simulink model "QD_V2"  (R2019a)
settings: Solver=ode4  StartTime=0  StopTime=10  FixedStep=0.001  RelTol=1e-3  EnableMultiTasking=on
model workspace (MAT data in the model file):
  ChStern = 20.5517740291
  CvStern = 205.517740291
  StartTime = '0'
  StopTime = '100'
  c = 0
  deltaControlled = 0
  deltaH = [0 0.02 0.04 0.06 0.08 0.1 0.12 0.14 0.16 0.18 0.2 0.22 0.24 0.26 0.28 0.3 0.32 0.34 0.36 0.38 0.4 0.42 0.44 0.46 0.48 0.5 0.52 0.54 0.56 0.58 0.6 0.62 0.64 0.66 0.68 0.7 0.72 0.74 0.76 0.78 0.8 0.82 0.84 0.86 0.88 0.9 0.92 0.94 0.96 0.98 1 1.02 1.04 1.06 1.08 1.1 1.12 1.14 1.16 1.18 1.2 1.22 1.24 1.26 1.28 1.3 1.32 1.34 1.36 1.38 1.4 1.42 1.44 1.46 1.48 1.5 1.52 1.54 1.56 1.58 1.6 1.62 1.64 1.66 1.68 1.7 1.72 1.74 1.76 1.78 1.8 1.82 1.84 1.86 1.88 1.9 1.92 1.94 1.96 1.98 2 2.02 2.04 2.06 2.08 2.1 2.12 2.14 2.16 2.18 2.2 2.22 2.24 2.26 2.28 2.3 2.32 2.34 2.36 2.38 2.4 2.42 2.44 2.46 2.48 2.5 2.52 2.54 2.56 2.58 2.6 2.62 2.64 2.66 2.68 2.7 2.72 2.74 2.76 2.78 2.8 2.82 2.84 2.86 2.88 2.9 2.92 2.94 2.96 2.98 3 3.02 3.04 3.06 3.08 3.1 3.12 3.14 3.16 3.18 3.2 3.22 3.24 3.26 3.28 3.3 3.32 3.34 3.36 3.38 3.4 3.42 3.44 3.46 3.48 3.5 3.52 3.54 3.56 3.58 3.6 3.62 3.64 3.66 3.68 3.7 3.72 3.74 3.76 3.78 3.8 3.82 3.84 3.86 3.88 3.9 3.92 3.94 3.96 3.98 4 4.02 4.04 4.06 4.08 4.1 4.12 4.14 4.16 4.18 4.2 4.22 4.24 4.26 4.28 4.3 4.32 4.34 4.36 4.38 4.4 4.42 4.44 4.46 4.48 4.5 4.52 4.54 4.56 4.58 4.6 4.62 4.64 4.66 4.68 4.7 4.72 4.74 4.76 4.78 4.8 4.82 4.84 4.86 4.88 4.9 4.92 4.94 4.96 4.98 5 5.02 5.04 5.06 5.08 5.1 5.12 5.14 5.16 5.18 5.2 5.22 5.24 5.26 5.28 5.3 5.32 5.34 5.36 5.38 5.4 5.42 5.44 5.46 5.48 5.5 5.52 5.54 5.56 5.58 5.6 5.62 5.64 5.66 5.68 5.7 5.72 5.74 5.76 5.78 5.8 5.82 5.84 5.86 5.88 5.9 5.92 5.94 5.96 5.98 6]
  g = 9.81
  is = 16
  lh = 1.45
  lv = 1.35
  m = 1550
  mDivTheta = 0.553571428571
  rSoll = 1
  theta = 2800
  v = 50
  x0 = 0
libraries: simulink x1
settings Model: Creator=tmonn  LastModifiedBy=Felix
settings DataIOCC: ExternalInput=c  ReturnWorkspaceOutputs=off
settings OptimizationCC: LifeSpan=inf
settings DebuggingCC: UnderspecifiedInitializationDetection=Classic  MergeDetectMultiDrivingBlocksExec=none  SFUnexpectedBacktrackingDiag=warning  SFNoUnconditionalDefaultTransitionDiag=warning  SFExecutionAtInitializationDiag=none  UnderSpecifiedDimensionMsg=warning  ArithmeticOperatorsInVariantConditions=warning
settings SFSimCC: SimUseLocalCustomCode=off
settings RTWCC: RTWUseLocalCustomCode=off
settings CodeAppCC: StateflowObjectComments=on
settings GRTTargetCC: TargetLangStandard=C89/C90 (ANSI)  GeneratePreprocessorConditionals=Disable all
settings ConfigComp: CovMetricSettings=dw  CovHtmlReporting=on  CovSaveCumulativeToWorkspaceVar=on  CovSaveSingleToWorkspaceVar=on  CovExternalEMLEnable=off

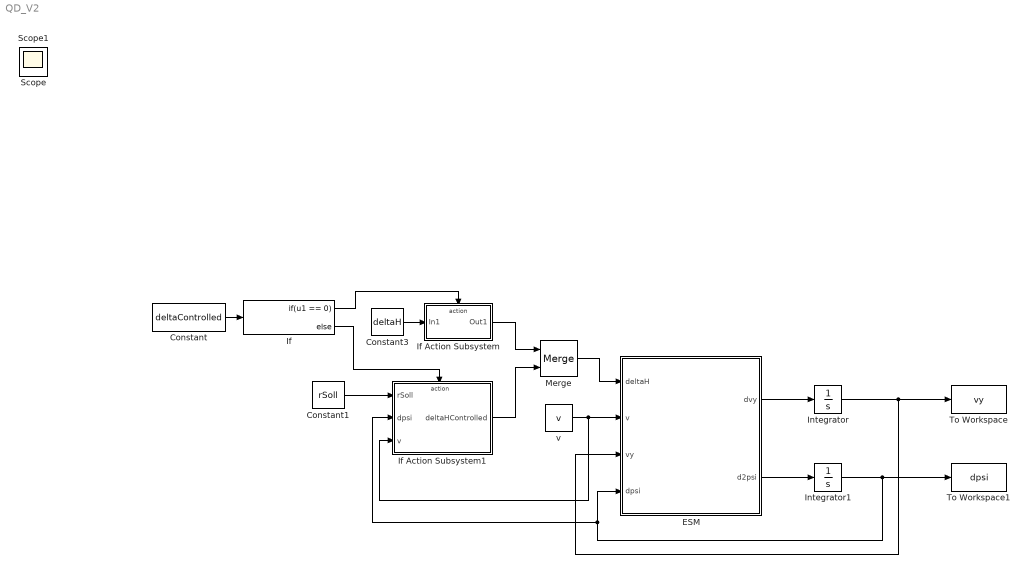
== system QD_V2 ==
  Constant : Constant  Value=deltaControlled
  Constant1 : Constant  Value=rSoll
  Constant3 : Constant  Value=deltaH
  ESM : Subsystem
  If : If  IfExpression=u1 == 0
  If Action Subsystem : Subsystem  TreatAsAtomicUnit=on
  If Action Subsystem1 : Subsystem  TreatAsAtomicUnit=on
  Integrator : Integrator
  Integrator1 : Integrator
  Merge : Merge  AllowUnequalInputPortWidths=on
  To Workspace : ToWorkspace  VariableName=vy  SaveFormat=Timeseries  SampleTime=-1
  To Workspace1 : ToWorkspace  VariableName=dpsi  SaveFormat=Timeseries  SampleTime=-1
  v : Constant  Value=v
  Scope : Scope
  Scope1 : Scope
  wires:
  ESM/1(dvy) -> Integrator/1
  ESM/2(d2psi) -> Integrator1/1
  Integrator/1 -> To Workspace/1, ESM/3(vy)
  If Action Subsystem/1(Out1) -> Merge/1
  Constant1/1 -> If Action Subsystem1/1(rSoll)
  If Action Subsystem1/1(deltaHControlled) -> Merge/2
  If/1 -> If Action Subsystem/Action
  If/2 -> If Action Subsystem1/Action
  Constant/1 -> If/1
  Merge/1 -> ESM/1(deltaH)
  Constant3/1 -> If Action Subsystem/1(In1)
  Integrator1/1 -> If Action Subsystem1/2(dpsi), ESM/4(dpsi), To Workspace1/1
  v/1 -> If Action Subsystem1/3(v), ESM/2(v)

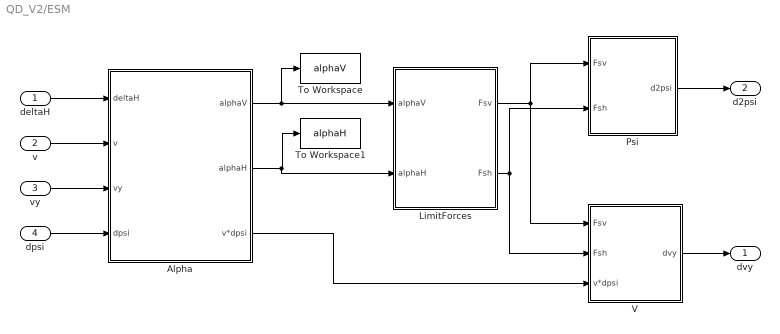
== system QD_V2/ESM ==
  deltaH : Inport
  v : Inport  Port=2
  vy : Inport  Port=3
  dpsi : Inport  Port=4
  Alpha : Subsystem
  LimitForces : Subsystem
  Psi : Subsystem
  To Workspace : ToWorkspace  VariableName=alphaV  SaveFormat=Timeseries  SampleTime=-1
  To Workspace1 : ToWorkspace  VariableName=alphaH  SaveFormat=Timeseries  SampleTime=-1
  V : Subsystem
  dvy : Outport
  d2psi : Outport  Port=2
  wires:
  deltaH/1 -> Alpha/1(deltaH)
  Alpha/1(alphaV) -> LimitForces/1(alphaV), To Workspace/1
  Alpha/2(alphaH) -> LimitForces/2(alphaH), To Workspace1/1
  v/1 -> Alpha/2(v)
  vy/1 -> Alpha/3(vy)
  dpsi/1 -> Alpha/4(dpsi)
  Psi/1(d2psi) -> d2psi/1
  V/1(dvy) -> dvy/1
  Alpha/3(v*dpsi) -> V/3(v*dpsi)
  LimitForces/2(Fsh) -> Psi/2(Fsh), V/2(Fsh)
  LimitForces/1(Fsv) -> V/1(Fsv), Psi/1(Fsv)

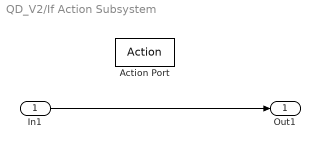
== system QD_V2/If Action Subsystem ==
  In1 : Inport
  Action Port : ActionPort  ActionPortLabel=if(u1 == 0)
  Out1 : Outport
  wires:
  In1/1 -> Out1/1

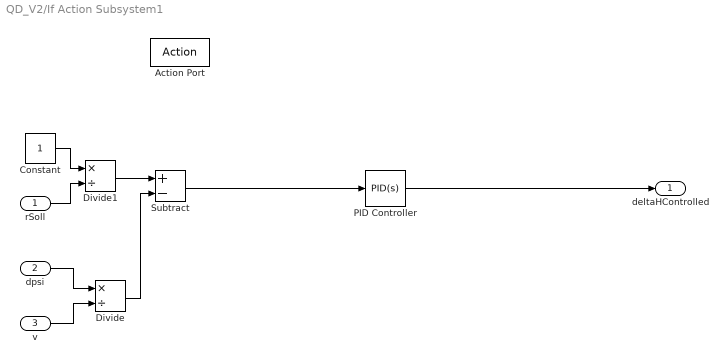
== system QD_V2/If Action Subsystem1 ==
  rSoll : Inport
  dpsi : Inport  Port=2
  v : Inport  Port=3
  Action Port : ActionPort  ActionPortLabel=else
  Constant : Constant
  Divide : Product  Inputs=*/
  Divide1 : Product  Inputs=*/
  PID Controller : simulink/Continuous/PID Controller  Controller=PID  Form=Parallel  TimeDomain=Continuous-time  SampleTime=-1  IntegratorMethod=Forward Euler  FilterMethod=Forward Euler  ControllerParametersSource=internal  P=1  I=1  D=0  UseFilter=on  N=100  TunerSelectOption=Transfer Function Based (PID Tuner App)  InitialConditionSource=internal  InitialConditionForIntegrator=0  InitialConditionForFilter=0  DifferentiatorICPrevScaledInput=0  ExternalReset=none  TrackingMode=off  Kt=1  LimitOutput=off  UpperSaturationLimit=inf  LowerSaturationLimit=-inf  LinearizeAsGain=on  AntiWindupMode=none  Kb=1  POutMin=[]  POutMax=[]  IOutMin=[]  IOutMax=[]  DOutMin=[]  DOutMax=[]  NOutMin=[]  NOutMax=[]  SumOutMin=[]  SumOutMax=[]  SaturationOutMin=[]  SaturationOutMax=[]  PParamMin=[]  PParamMax=[]  IParamMin=[]  IParamMax=[]  DParamMin=[]  DParamMax=[]  NParamMin=[]  NParamMax=[]  KbParamMin=[]  KbParamMax=[]  KtParamMin=[]  KtParamMax=[]  KbOutMin=[]  KbOutMax=[]  KtOutMin=[]  KtOutMax=[]  IntegratorOutMin=[]  IntegratorOutMax=[]  FilterOutMin=[]  FilterOutMax=[]  SumI1OutMin=[]  SumI1OutMax=[]  SumI2OutMin=[]  SumI2OutMax=[]  SumI3OutMin=[]  SumI3OutMax=[]  SumI4OutMin=[]  SumI4OutMax=[]  SumDOutMin=[]  SumDOutMax=[]  DifferentiatorOutMin=[]  DifferentiatorOutMax=[]  FilterDiffOutCoefMin=[]  FilterDiffOutCoefMax=[]  ReciprocalOutMin=[]  ReciprocalOutMax=[]  SumDenOutMin=[]  SumDenOutMax=[]  SumNumOutMin=[]  SumNumOutMax=[]  DivideOutMin=[]  DivideOutMax=[]  IntegratorContinuousStateAttributes=''  IntegratorStateMustResolveToSignalObject=off  IntegratorRTWStateStorageClass=Auto  FilterContinuousStateAttributes=''  FilterStateMustResolveToSignalObject=off  FilterRTWStateStorageClass=Auto  ParallelPVariant=InternalParameters  IdealPVariant=Disabled  IVariant=InternalParameters  DVariant=InternalParameters  IntegratorVariant=Continuous  SatVariant=Disabled  AWVariant=Passthrough  PCopyVariant=Disabled  TRVariant=Disabled  FdbkBlocksVariant=Forward  IdealPFdbkVariant=Disabled  SatFdbkVariant=Disabled  DerivativeFilterVariant=ContFilter  NVariant=InternalParameters  NCopyVariant=Disabled  FilterICVariant=InternalICsFilter  IntegratorICVariant=InternalICs  ExternalResetVariant=Disabled  TRSumVariant=Passthrough  SumFdbkVariant=Disabled  SumVariant=Sum_PID
  Subtract : Sum  Inputs=+-
  deltaHControlled : Outport
  wires:
  Divide/1 -> Subtract/2
  Constant/1 -> Divide1/1
  rSoll/1 -> Divide1/2
  Divide1/1 -> Subtract/1
  v/1 -> Divide/2
  dpsi/1 -> Divide/1
  Subtract/1 -> PID Controller/1
  PID Controller/1 -> deltaHControlled/1

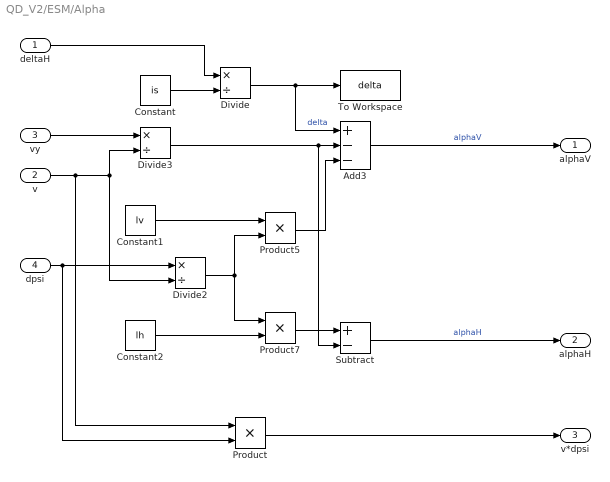
== system QD_V2/ESM/Alpha ==
  deltaH : Inport
  v : Inport  Port=2
  vy : Inport  Port=3
  dpsi : Inport  Port=4
  Add3 : Sum  Inputs=+--
  Constant : Constant  Value=is
  Constant1 : Constant  Value=lv
  Constant2 : Constant  Value=lh
  Divide : Product  Inputs=*/
  Divide2 : Product  Inputs=*/
  Divide3 : Product  Inputs=*/
  Product : Product
  Product5 : Product
  Product7 : Product
  Subtract : Sum  Inputs=+-
  To Workspace : ToWorkspace  VariableName=delta  SaveFormat=Timeseries  SampleTime=-1
  alphaV : Outport
  alphaH : Outport  Port=2
  v*dpsi : Outport  Port=3
  wires:
  Divide3/1 -> Subtract/2, Add3/2
  Divide2/1 -> Product7/1, Product5/2
  dpsi/1 -> Product/2, Divide2/1
  vy/1 -> Divide3/1
  Product5/1 -> Add3/3
  Constant1/1 -> Product5/1
  Constant2/1 -> Product7/2
  Product7/1 -> Subtract/1
  Divide/1 -> Add3/1, To Workspace/1  "delta"
  deltaH/1 -> Divide/1
  Constant/1 -> Divide/2
  Product/1 -> v*dpsi/1
  v/1 -> Product/1, Divide2/2, Divide3/2
  Add3/1 -> alphaV/1  "alphaV"
  Subtract/1 -> alphaH/1  "alphaH"

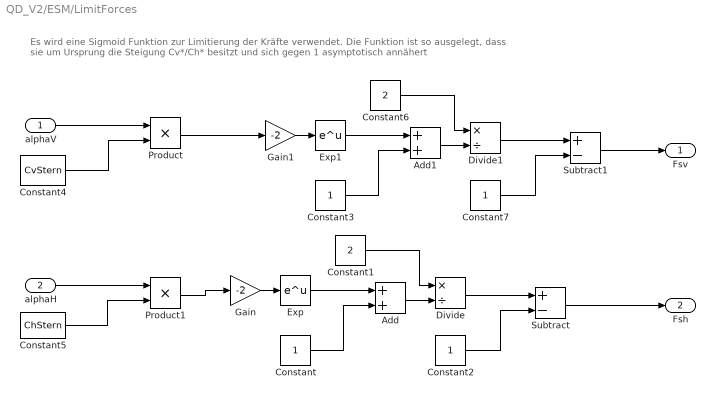
== system QD_V2/ESM/LimitForces ==
  note: Es wird eine Sigmoid Funktion zur Limitierung der Kräfte verwendet. Die Funktion ist so ausgelegt, dass sie um Ursprung die Steigung Cv*/Ch* besitzt
      | und sich gegen 1 asymptotisch annähert
  alphaV : Inport
  alphaH : Inport  Port=2
  Add : Sum
  Add1 : Sum
  Constant{,2..3,7} (4 alike) : Constant
  Constant1 : Constant  Value=2
  Constant4 : Constant  Value=CvStern
  Constant5 : Constant  Value=ChStern
  Constant6 : Constant  Value=2
  Divide : Product  Inputs=*/
  Divide1 : Product  Inputs=*/
  Exp : Math  SaturateOnIntegerOverflow=on
  Exp1 : Math  SaturateOnIntegerOverflow=on
  Gain : Gain  Gain=-2
  Gain1 : Gain  Gain=-2
  Product : Product
  Product1 : Product
  Subtract : Sum  Inputs=+-
  Subtract1 : Sum  Inputs=+-
  Fsv : Outport
  Fsh : Outport  Port=2
  wires:
  Constant4/1 -> Product/2
  Constant5/1 -> Product1/2
  Exp/1 -> Add/1
  Gain/1 -> Exp/1
  Constant/1 -> Add/2
  Add/1 -> Divide/2
  Constant1/1 -> Divide/1
  Divide/1 -> Subtract/1
  Constant2/1 -> Subtract/2
  Constant6/1 -> Divide1/1
  Add1/1 -> Divide1/2
  Gain1/1 -> Exp1/1
  Divide1/1 -> Subtract1/1
  Constant7/1 -> Subtract1/2
  Constant3/1 -> Add1/2
  Exp1/1 -> Add1/1
  Product1/1 -> Gain/1
  Subtract/1 -> Fsh/1
  Product/1 -> Gain1/1
  Subtract1/1 -> Fsv/1
  alphaH/1 -> Product1/1
  alphaV/1 -> Product/1

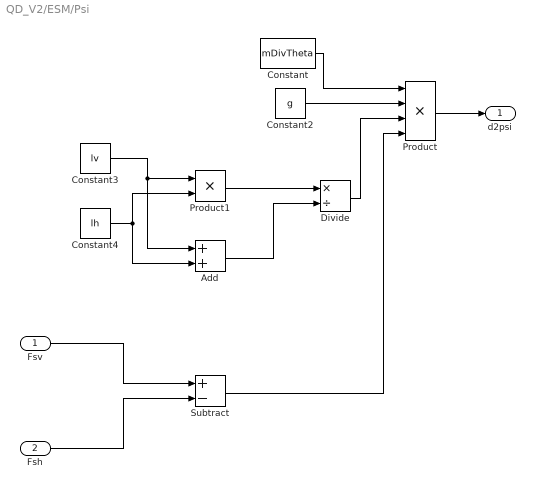
== system QD_V2/ESM/Psi ==
  Fsv : Inport
  Fsh : Inport  Port=2
  Add : Sum
  Constant : Constant  Value=mDivTheta
  Constant2 : Constant  Value=g
  Constant3 : Constant  Value=lv
  Constant4 : Constant  Value=lh
  Divide : Product  Inputs=*/
  Product : Product  Inputs=4
  Product1 : Product
  Subtract : Sum  Inputs=+-
  d2psi : Outport
  wires:
  Constant2/1 -> Product/2
  Divide/1 -> Product/3
  Product1/1 -> Divide/1
  Add/1 -> Divide/2
  Constant3/1 -> Add/1, Product1/1
  Constant4/1 -> Product1/2, Add/2
  Product/1 -> d2psi/1
  Subtract/1 -> Product/4
  Fsv/1 -> Subtract/1
  Fsh/1 -> Subtract/2
  Constant/1 -> Product/1

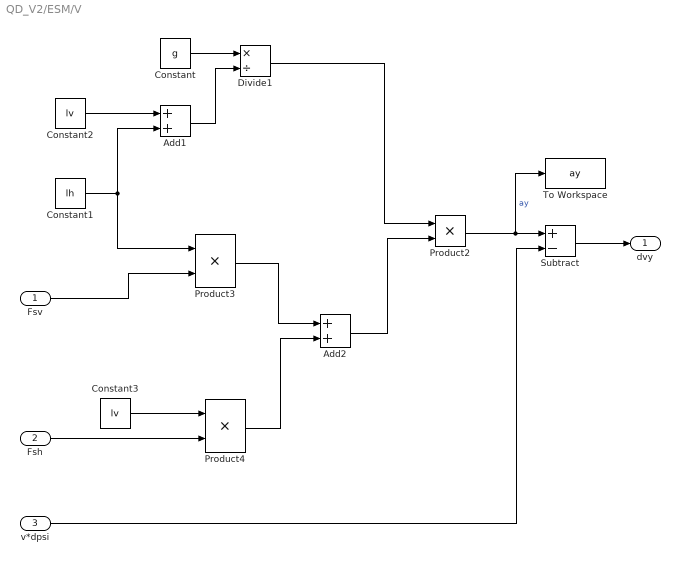
== system QD_V2/ESM/V ==
  Fsv : Inport
  Fsh : Inport  Port=2
  v*dpsi : Inport  Port=3
  Add1 : Sum
  Add2 : Sum
  Constant : Constant  Value=g
  Constant1 : Constant  Value=lh
  Constant2 : Constant  Value=lv
  Constant3 : Constant  Value=lv
  Divide1 : Product  Inputs=*/
  Product2 : Product
  Product3 : Product
  Product4 : Product
  Subtract : Sum  Inputs=+-
  To Workspace : ToWorkspace  VariableName=ay  SaveFormat=Timeseries  SampleTime=-1
  dvy : Outport
  wires:
  Add1/1 -> Divide1/2
  Divide1/1 -> Product2/1
  Add2/1 -> Product2/2
  Constant1/1 -> Add1/2, Product3/1
  Product3/1 -> Add2/1
  Product4/1 -> Add2/2
  Fsv/1 -> Product3/2
  Fsh/1 -> Product4/2
  Constant/1 -> Divide1/1
  Constant2/1 -> Add1/1
  Constant3/1 -> Product4/1
  v*dpsi/1 -> Subtract/2
  Subtract/1 -> dvy/1
  Product2/1 -> Subtract/1, To Workspace/1  "ay"
